simulink library "xblocks_library_pfbs"  (Simulink 7.6)
settings: Solver=ode45  SolverMode=SingleTasking  StartTime=0.0  StopTime=10.0  RelTol=1e-3
libraries: xbsIndex_r4 x151
(part 1 of 2)
settings Model: Creator=mdexter  LastModifiedBy=Glenn

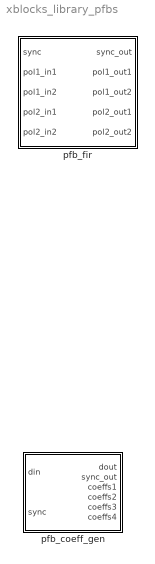
== system xblocks_library_pfbs ==
  pfb_coeff_gen : Subsystem  mask(pfb_coeff_gen){PFBSize=6, CoeffBitWidth=8, TotalTaps=4, CoeffDistMem=0, WindowType=hamming, bram_latency=2, n_inputs=0, nput=0, fwidth=1}
      mask prompts: PFBSize "Size of PFB: (2^? pnts)"; CoeffBitWidth "Bitwidth of Coefficients:"; TotalTaps "Total Number of Taps:"; CoeffDistMem "Implement Coeff Gen in Distributed Memory"; WindowType "Windowing Function:"; bram_latency "BRAM Latency"; n_inputs "Number of Simultaneous Inputs: (2^?)"; nput "This is input number:"; fwidth "Bin Width (normal=1)"
      mask init:
      | config.source = str2func('pfb_coeff_gen_init_xblock');
      | config.toplevel = gcb;
      | config.depend = get_dependlist('pfb_coeff_gen');
      | set_param(gcb,'LinkStatus','inactive');
      | xBlock(config, {config.toplevel, ...
      |     PFBSize, ...
      |     CoeffBitWidth, ...
      |     TotalTaps, ...
      |     CoeffDistMem, ...
      |     WindowType, ...
      |     bram_latency, ...
      |     n_inputs, ...
      |     nput, ...
      |     fwidth});
      settings: AttributesFormatString=PFBSize=6, n_inputs=0, taps=4
  pfb_fir : Subsystem  mask(pfb_fir){PFBSize=5, TotalTaps=2, WindowType=hamming, n_inputs=1, MakeBiplex=on, BitWidthIn=8, BitWidthOut=18, CoeffBitWidth=18, CoeffDistMem=off, add_latency=1, mult_latency=2, bram_latency=2, quantization=Round  (unbiased: +/- Inf), fwidth=1, specify_mult=off, mult_spec=[2                                      2], oversample_factor=0, oversample_index=0}
      mask prompts: PFBSize "Size of PFB: (2^? pnts)"; TotalTaps "Total Number of Taps:"; WindowType "Windowing Function:"; n_inputs "Number of Simultaneous Inputs: (2^?)"; MakeBiplex "Make Biplex"; BitWidthIn "Input Bitwidth:"; BitWidthOut "Output Bitwidth:"; CoeffBitWidth "Coefficient Bitwidth:"; CoeffDistMem "Use Distributed Memory for Coeffs"; add_latency "Add Latency"; mult_latency "Mult Latency"; bram_latency "BRAM Latency"; quantization "Quantization Behavior"; fwidth "Bin Width Scaling (normal=1)"; specify_mult "Specify multiplier use (behavioral if not specified)"; mult_spec "Multiplier specification (0=core, 1=embedded, 2=behavioural) (left=1st tap)"; oversample_factor "Oversample factor (normal=1)"; oversample_index "Oversample index (0 upto oversample factor)"
      mask init:
      | config.source = str2func('pfb_fir_init_xblock');
      | config.toplevel = gcb;
      | config.depend = get_dependlist('pfb_fir');
      | set_param(gcb,'LinkStatus','inactive');
      | xBlock(config,{config.toplevel, ...
      |     'PFBSize', PFBSize, ...
      |     'TotalTaps', TotalTaps, ...
      |     'WindowType', WindowType, ...
      |     'n_inputs', n_inputs, ...
      |     'MakeBiplex', MakeBiplex, ...
      |     'BitWidthIn', BitWidthIn, ...
      |     'BitWidthOut', BitWidthOut, ...
      |     'CoeffBitWidth', CoeffBitWidth, ...
      |     'CoeffDistMem', CoeffDistMem, ...
      |     'add_latency', add_latency, ...
      |     'mult_latency', mult_latency, ...
      |     'bram_latency', bram_latency, ...
      |     'quantization', quantization, ...
      |     'fwidth', fwidth,...
      |     'specify_mult', specify_mult,...
      |     'mult_spec', mult_spec,...
      |     'oversample_factor', oversample_factor,...
      |     'oversample_index', oversample_index});
      settings: AttributesFormatString=taps=2, add_latency=1
      mask Help: eval('xlWeb(''http://casper.berkeley.edu/wiki/Pfb_fir'')')
      mask StyleString: edit,edit,popup(bartlett|barthannwin|blackman|blackmanharris|bohamwin|chebwin|flattopwin|gausswin|hamming|hann|kaiser|nuttallwin|parzenwin|rectwin|tukeywin|triang|userwindow),edit,checkbox,edit,edit,edit,checkbox,edit,edit,edit,popup(Truncate|Round  (unbiased: +/- Inf)|Round  (unbiased: Even Values)),edit,checkbox,edit,edit,edit
      mask CallbackString:
      | |%num_taps = eval(get_param(gcb, 'TotalTaps'));
      | %old_vec = eval(get_param(gcb, 'mult_spec'));
      | 
      | %vec = 2.*ones(1,num_taps);
      | %old_size = length(old_vec);
      | 
      | %if(old_size <= num_taps),
      | %   new_size = old_size;
      | %else,
      | %    new_size = num_taps;
      | %end
      | 
      | %for n = 1:new_size, vec(n) = old_vec(n); end
      | %set_param(gcb, 'mult_spec', mat2str(vec));||||||||||||%num_taps = eval(get_param(gcb, 'TotalTaps'));
      | %old_vec = eval(get_param(gcb, 'mult_spec'));
      | 
      | %vec = 2.*ones(1,num_taps);
      | %old_size = length(old_vec);
      | 
      | %if(old_size <= num_taps),
      | %    new_size = old_size;
      | %else,
      | %    new_size = num_taps;
      | %end
      | 
      | %for n = 1:new_size, vec(n) = old_vec(n); end
      | %set_param(gcb, 'mult_spec', mat2str(vec));|%specify_mult = get_param(gcb,'specify_mult');
      | %if( strcmp(specify_mult,'off')),
      | %    set_param(gcb, 'MaskEnables', {'on','on','on','on','on','on','on','on','on','on','on','on','on','on','on','off'});
      | %else
      | %    set_param(gcb, 'MaskEnables', {'on','on','on','on','on','on','on','on','on','on','on','on','on','on','on','on'});
      | %end
      | 
      | |%specify_mult = get_param(gcb,'specify_mult');
      | %if( strcmp(specify_mult,'off')),
      | %    set_param(gcb, 'MaskEnables', {'on','on','on','on','on','on','on','on','on','on','on','on','on','on','on','off'});
      | %else
      | %    set_param(gcb, 'MaskEnables', {'on','on','on','on','on','on','on','on','on','on','on','on','on','on','on','on'});
      | %end
      | 
      | ||

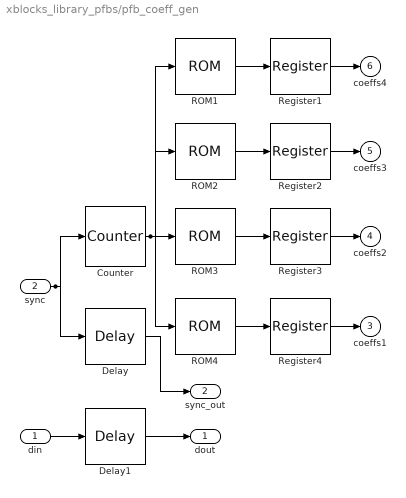
== system xblocks_library_pfbs/pfb_coeff_gen ==
  din : Inport
  sync : Inport  Port=2
  Counter : xbsIndex_r4/Counter  cnt_type=Free Running  cnt_to=Inf  operation=Up  start_count=0  cnt_by_val=1  arith_type=Unsigned  n_bits=6  bin_pt=0  load_pin=off  rst=on  en=off  explicit_period=on  period=1  dbl_ovrd=off  use_behavioral_HDL=off  implementation=Fabric  use_rpm=on  block_type=counter
  Delay : xbsIndex_r4/Delay  en=off  latency=3  dbl_ovrd=off  reg_retiming=off  block_type=delay
  Delay1 : xbsIndex_r4/Delay  en=off  latency=3  dbl_ovrd=off  reg_retiming=off  block_type=delay
  ROM1 : xbsIndex_r4/ROM  depth=64  initVector=[-3.1185374660155e-018 -0.000630767340734862 -0.00127665235543742 -0.00194310743224035 -0.00263564676491746 -0.00335979233260294 -0.00412101838978196 -0.00492469476174935 -0.00577602925112446 -0.00668000946994591 -0.0076413444192915 -0.00866440614422574 -0.00975317179612738 -0.010911166437057 -0.0121414069217606 -0.0134463471921525 -0.0148278253166674 -0.0162870126027097 -0.0178243651045739 -0.0194395778416632 -0.0211315420326285 -0.022898305640208 -0.0247370375091149 -0.0266439953653345 -0.0286144979297191 -0.0306429013818577 -0.0327225803919297 -0.0348459139186967 -0.0370042759510287 -0.039188031348495 -0.0413865369136648 -0.0435881478049666 -0.0457802293743504 -0.0479491744886968 -0.0500804263680376 -0.0521585069473131 -0.0541670507417091 -0.0560888441687308 -0.0579058702531857 -0.0595993586143156 -0.0611498406075495 -0.0625372094668812 -0.0637407852678391 -0.0647393845055283 -0.0655113940574241 -0.0660348492765973 -0.0662875159379727 -0.0662469757381941 -0.0658907150287818 -0.0651962164426562 -0.0641410530558401 -0.0627029847093632 -0.0608600561011471 -0.0585906962440446 -0.0558738188743138 -0.0526889233846958 -0.0490161958479985 -0.0448366096907167 -0.0401320255717928 -0.0348852900191694 -0.0290803323763385 -0.0227022596126709 -0.0157374485549124 -0.00817363510287419]  distributed_mem=Block RAM  rst=off  init_reg=0  en=off  latency=2  arith_type="Signed  (2's comp)"  n_bits=8  bin_pt=7  dbl_ovrd=off  optimize=Area  use_rpm=on  block_type=sprom
  ROM2 : xbsIndex_r4/ROM  depth=64  initVector=[2.11605855357879e-017 0.00879274926085128 0.0182123008044376 0.0282646654074538 0.038954108579165 0.0502830880501052 0.0622521970115558 0.0748601134277915 0.0881035557207456 0.101977245102897 0.116473874808906 0.131584086449929 0.147296453686772 0.16359747338912 0.180471564418265 0.197901074140048 0.215866292743331 0.234345475407368 0.253314872329023 0.272748766588106 0.29261951979626 0.312897625441996 0.333551769811778 0.354548900334662 0.375854301166013 0.39743167579445 0.419243236425489 0.441249799865535 0.463410889601092 0.485684843740308 0.508028928457608 0.530399456557046 0.552751910746464 0.575041071192575 0.597221146906817 0.619245910493353 0.641068835774032 0.662643237790492 0.683922414671039 0.704859790839448 0.725409061034526 0.745524334603159 0.765160279525672 0.784272265630716 0.802816506457524 0.820750199226298 0.838031662382672 0.854620470189629 0.870477583849913 0.885565478653822 0.899848266661255 0.91329181444297 0.925863855424124 0.937534096393168 0.948274317761146 0.958058467180069 0.966862746154448 0.974665689306961 0.981448235987612 0.987193793945478 0.99188829481302 0.995520241184955 0.998080745106585 0.99956355782024]  distributed_mem=Block RAM  rst=off  init_reg=0  en=off  latency=2  arith_type="Signed  (2's comp)"  n_bits=8  bin_pt=7  dbl_ovrd=off  optimize=Area  use_rpm=on  block_type=sprom
  ROM3 : xbsIndex_r4/ROM  depth=64  initVector=[0.999965090652822 0.99928442696235 0.99752332509661 0.994686212352466 0.990780169959861 0.985814909149891 0.979802738401511 0.972758521996084 0.964699630043176 0.955645880174459 0.945619471135172 0.934644908534211 0.922748923044456 0.909960381374135 0.89631019035795 0.881831194543024 0.866558067669544 0.850527198468991 0.83377657122414 0.816345641554348 0.798275207907048 0.779607279251688 0.760384939485607 0.740652209072382 0.720453904442071 0.699835495689393 0.678842963110256 0.657522653119166 0.635921134089847 0.614085052658984 0.592060991028308 0.569895325793337 0.547634088817976 0.525322830662984 0.503006487062978 0.480729248931329 0.458534436355056 0.436464377022686 0.414560289507162 0.39286217180335 0.371408695495545 0.350237105904836 0.329383128539273 0.308880882141693 0.288762798600841 0.269059549961341 0.249799982737069 0.231011059700927 0.212717809291838 0.194943282747282 0.177708519036935 0.161032517640107 0.144932219176911 0.129422493870459 0.114516137785164 0.100223876754423 0.0865543778798294 0.0735142684536453 0.0611081621267689 0.0493386921159191 0.0382065512163987 0.0277105383606731 0.0178476114382339 0.0086129460689059]  distributed_mem=Block RAM  rst=off  init_reg=0  en=off  latency=2  arith_type="Signed  (2's comp)"  n_bits=8  bin_pt=7  dbl_ovrd=off  optimize=Area  use_rpm=on  block_type=sprom
  ROM4 : xbsIndex_r4/ROM  depth=64  initVector=[2.07187717402902e-017 -0.00799941722240988 -0.0153950696762068 -0.0221982159646857 -0.0284215259962463 -0.0340789940546858 -0.0391858485833677 -0.0437584591154741 -0.0478142407894676 -0.0513715568937888 -0.0544496198876778 -0.0570683913458442 -0.0592484812735286 -0.0610110472353188 -0.0623776937359413 -0.0633703722841764 -0.0640112825620935 -0.0643227751110339 -0.0643272559332322 -0.0640470933937545 -0.0635045277916038 -0.0627215839515021 -0.0617199871690848 -0.0605210828221477 -0.0591457599392603 -0.0576143789946302 -0.0559467041746632 -0.0541618403373513 -0.0522781748605462 -0.0503133245494637 -0.0482840877475476 -0.0462064017682173 -0.0440953057381763 -0.0419649089159751 -0.0398283645225593 -0.0376978490936883 -0.0355845473375377 -0.0334986424546007 -0.0314493118513142 -0.0294447281537699 -0.0274920654035405 -0.0255975102941681 -0.023766278284333 -0.0220026344022442 -0.0203099185354575 -0.0186905749812331 -0.017146186014759 -0.0156775092161722 -0.0142845182823737 -0.0129664470362087 -0.01172183633373 -0.0105485835600183 -0.00944399439543556 -0.0084048365272635 -0.00742739497645097 -0.0065075287056645 -0.00564072817301709 -0.00482217349572776 -0.00404679288952885 -0.00330932105286414 -0.00260435716978029 -0.00192642221186661 -0.00127001522759956 -0.000629668316944681]  distributed_mem=Block RAM  rst=off  init_reg=0  en=off  latency=2  arith_type="Signed  (2's comp)"  n_bits=8  bin_pt=7  dbl_ovrd=off  optimize=Area  use_rpm=on  block_type=sprom
  Register{1..4} (4 alike) : xbsIndex_r4/Register  init=0  rst=off  en=off  dbl_ovrd=off  block_type=register
  dout : Outport
  sync_out : Outport  Port=2
  coeffs1 : Outport  Port=3
  coeffs2 : Outport  Port=4
  coeffs3 : Outport  Port=5
  coeffs4 : Outport  Port=6
  wires:
  sync/1 -> Delay/1, Counter/1
  Counter/1 -> ROM1/1, ROM2/1, ROM3/1, ROM4/1
  Register1/1 -> coeffs4/1
  ROM1/1 -> Register1/1
  Register2/1 -> coeffs3/1
  ROM2/1 -> Register2/1
  Register3/1 -> coeffs2/1
  ROM3/1 -> Register3/1
  Register4/1 -> coeffs1/1
  ROM4/1 -> Register4/1
  Delay1/1 -> dout/1
  din/1 -> Delay1/1
  Delay/1 -> sync_out/1

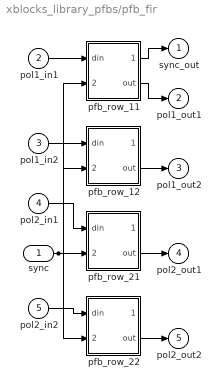
== system xblocks_library_pfbs/pfb_fir ==
  sync : Inport
  pol1_in1 : Inport  Port=2
  pol1_in2 : Inport  Port=3
  pol2_in1 : Inport  Port=4
  pol2_in2 : Inport  Port=5
  pfb_row_11 : Subsystem
  pfb_row_12 : Subsystem
  pfb_row_21 : Subsystem
  pfb_row_22 : Subsystem
  sync_out : Outport
  pol1_out1 : Outport  Port=2
  pol1_out2 : Outport  Port=3
  pol2_out1 : Outport  Port=4
  pol2_out2 : Outport  Port=5
  wires:
  sync/1 -> pfb_row_22/2(sync), pfb_row_21/2(sync), pfb_row_12/2(sync), pfb_row_11/2(sync)
  pfb_row_22/2(out) -> pol2_out2/1
  pol2_in2/1 -> pfb_row_22/1(din)
  pfb_row_21/2(out) -> pol2_out1/1
  pol2_in1/1 -> pfb_row_21/1(din)
  pfb_row_12/2(out) -> pol1_out2/1
  pol1_in2/1 -> pfb_row_12/1(din)
  pfb_row_11/2(out) -> pol1_out1/1
  pfb_row_11/1(sync_out) -> sync_out/1
  pol1_in1/1 -> pfb_row_11/1(din)

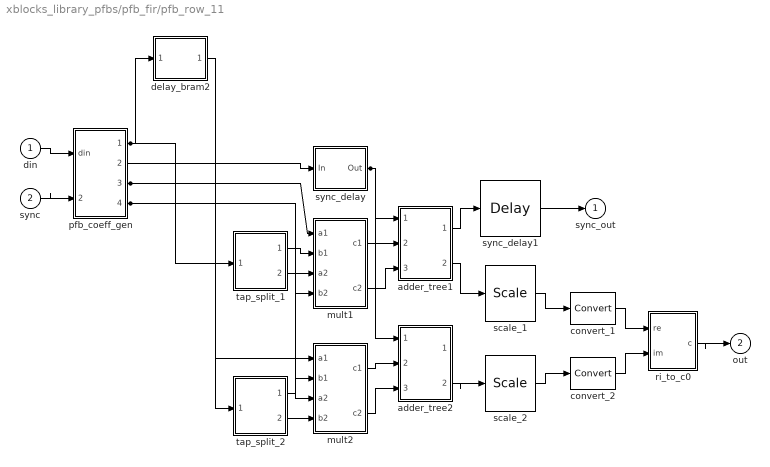
== system xblocks_library_pfbs/pfb_fir/pfb_row_11 ==
  din : Inport
  sync : Inport  Port=2
  adder_tree1 : Subsystem
  adder_tree2 : Subsystem
  convert_1 : xbsIndex_r4/Convert  arith_type="Signed  (2's comp)"  n_bits=18  bin_pt=17  quantization="Round  (unbiased: +/- Inf)"  overflow=Saturate  en=off  latency=2  dbl_ovrd=off  pipeline=on  block_type=convert
  convert_2 : xbsIndex_r4/Convert  arith_type="Signed  (2's comp)"  n_bits=18  bin_pt=17  quantization="Round  (unbiased: +/- Inf)"  overflow=Saturate  en=off  latency=2  dbl_ovrd=off  pipeline=on  block_type=convert
  delay_bram2 : Subsystem
  mult1 : Subsystem
  mult2 : Subsystem
  pfb_coeff_gen : Subsystem
      settings: AttributesFormatString=PFBSize=5, n_inputs=1, taps=2
  ri_to_c0 : Subsystem
  scale_1 : xbsIndex_r4/Scale  scale_factor=-2  dbl_ovrd=off  block_type=scale
  scale_2 : xbsIndex_r4/Scale  scale_factor=-2  dbl_ovrd=off  block_type=scale
  sync_delay : Subsystem
  sync_delay1 : xbsIndex_r4/Delay  en=off  latency=2  dbl_ovrd=off  reg_retiming=off  block_type=delay
  tap_split_1 : Subsystem
      settings: AttributesFormatString=Fix_8_7
  tap_split_2 : Subsystem
      settings: AttributesFormatString=Fix_8_7
  sync_out : Outport
  out : Outport  Port=2
  wires:
  pfb_coeff_gen/1(dout) -> tap_split_1/1(inport), delay_bram2/1(din_1_1)
  pfb_coeff_gen/3(coeffs1) -> mult2/1(a1), mult1/1(a1)
  pfb_coeff_gen/4(coeffs2) -> mult2/3(a2), mult1/3(a2)
  sync_delay/1(Out) -> adder_tree2/1(sync), adder_tree1/1(sync)
  ri_to_c0/1(c) -> out/1
  convert_2/1 -> ri_to_c0/2(im)
  convert_1/1 -> ri_to_c0/1(re)
  scale_2/1 -> convert_2/1
  adder_tree2/2(dout) -> scale_2/1
  mult2/2(c2) -> adder_tree2/3(din_2)
  mult2/1(c1) -> adder_tree2/2(din_1)
  tap_split_2/2(outport2) -> mult2/4(b2)
  tap_split_1/2(outport2) -> mult2/2(b1)
  sync_delay1/1 -> sync_out/1
  adder_tree1/1(sync_out) -> sync_delay1/1
  scale_1/1 -> convert_1/1
  adder_tree1/2(dout) -> scale_1/1
  mult1/2(c2) -> adder_tree1/3(din_2)
  mult1/1(c1) -> adder_tree1/2(din_1)
  tap_split_2/1(outport1) -> mult1/4(b2)
  tap_split_1/1(outport1) -> mult1/2(b1)
  delay_bram2/1(dout_1_1) -> tap_split_2/1(inport)
  pfb_coeff_gen/2(sync_out) -> sync_delay/1(In)
  sync/1 -> pfb_coeff_gen/2(sync)
  din/1 -> pfb_coeff_gen/1(din)

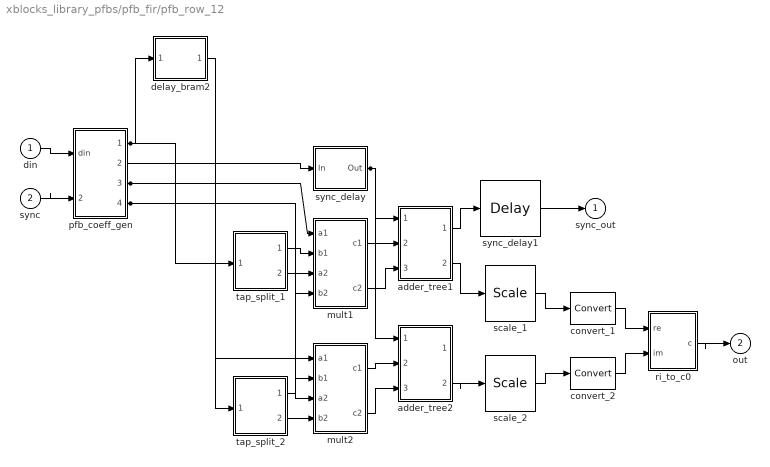
== system xblocks_library_pfbs/pfb_fir/pfb_row_12 ==
  din : Inport
  sync : Inport  Port=2
  adder_tree1 : Subsystem
  adder_tree2 : Subsystem
  convert_1 : xbsIndex_r4/Convert  arith_type="Signed  (2's comp)"  n_bits=18  bin_pt=17  quantization="Round  (unbiased: +/- Inf)"  overflow=Saturate  en=off  latency=2  dbl_ovrd=off  pipeline=on  block_type=convert
  convert_2 : xbsIndex_r4/Convert  arith_type="Signed  (2's comp)"  n_bits=18  bin_pt=17  quantization="Round  (unbiased: +/- Inf)"  overflow=Saturate  en=off  latency=2  dbl_ovrd=off  pipeline=on  block_type=convert
  delay_bram2 : Subsystem
  mult1 : Subsystem
  mult2 : Subsystem
  pfb_coeff_gen : Subsystem
      settings: AttributesFormatString=PFBSize=5, n_inputs=1, taps=2
  ri_to_c0 : Subsystem
  scale_1 : xbsIndex_r4/Scale  scale_factor=-2  dbl_ovrd=off  block_type=scale
  scale_2 : xbsIndex_r4/Scale  scale_factor=-2  dbl_ovrd=off  block_type=scale
  sync_delay : Subsystem
  sync_delay1 : xbsIndex_r4/Delay  en=off  latency=2  dbl_ovrd=off  reg_retiming=off  block_type=delay
  tap_split_1 : Subsystem
      settings: AttributesFormatString=Fix_8_7
  tap_split_2 : Subsystem
      settings: AttributesFormatString=Fix_8_7
  sync_out : Outport
  out : Outport  Port=2
  wires:
  pfb_coeff_gen/1(dout) -> tap_split_1/1(inport), delay_bram2/1(din_1_1)
  pfb_coeff_gen/3(coeffs1) -> mult2/1(a1), mult1/1(a1)
  pfb_coeff_gen/4(coeffs2) -> mult2/3(a2), mult1/3(a2)
  sync_delay/1(Out) -> adder_tree2/1(sync), adder_tree1/1(sync)
  ri_to_c0/1(c) -> out/1
  convert_2/1 -> ri_to_c0/2(im)
  convert_1/1 -> ri_to_c0/1(re)
  scale_2/1 -> convert_2/1
  adder_tree2/2(dout) -> scale_2/1
  mult2/2(c2) -> adder_tree2/3(din_2)
  mult2/1(c1) -> adder_tree2/2(din_1)
  tap_split_2/2(outport2) -> mult2/4(b2)
  tap_split_1/2(outport2) -> mult2/2(b1)
  sync_delay1/1 -> sync_out/1
  adder_tree1/1(sync_out) -> sync_delay1/1
  scale_1/1 -> convert_1/1
  adder_tree1/2(dout) -> scale_1/1
  mult1/2(c2) -> adder_tree1/3(din_2)
  mult1/1(c1) -> adder_tree1/2(din_1)
  tap_split_2/1(outport1) -> mult1/4(b2)
  tap_split_1/1(outport1) -> mult1/2(b1)
  delay_bram2/1(dout_1_1) -> tap_split_2/1(inport)
  pfb_coeff_gen/2(sync_out) -> sync_delay/1(In)
  sync/1 -> pfb_coeff_gen/2(sync)
  din/1 -> pfb_coeff_gen/1(din)

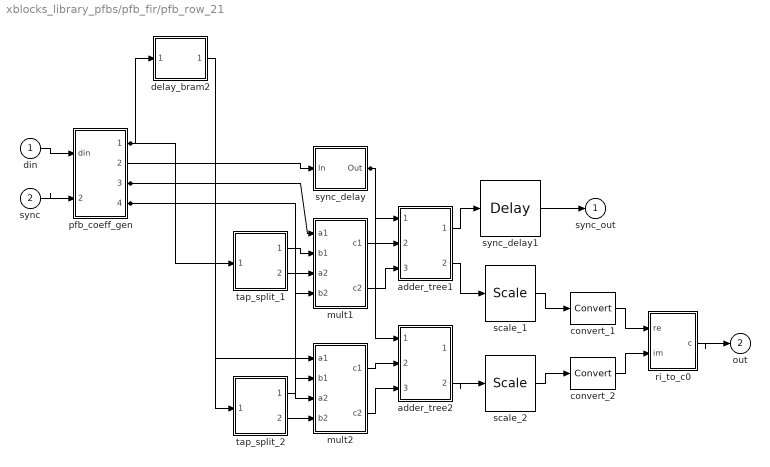
== system xblocks_library_pfbs/pfb_fir/pfb_row_21 ==
  din : Inport
  sync : Inport  Port=2
  adder_tree1 : Subsystem
  adder_tree2 : Subsystem
  convert_1 : xbsIndex_r4/Convert  arith_type="Signed  (2's comp)"  n_bits=18  bin_pt=17  quantization="Round  (unbiased: +/- Inf)"  overflow=Saturate  en=off  latency=2  dbl_ovrd=off  pipeline=on  block_type=convert
  convert_2 : xbsIndex_r4/Convert  arith_type="Signed  (2's comp)"  n_bits=18  bin_pt=17  quantization="Round  (unbiased: +/- Inf)"  overflow=Saturate  en=off  latency=2  dbl_ovrd=off  pipeline=on  block_type=convert
  delay_bram2 : Subsystem
  mult1 : Subsystem
  mult2 : Subsystem
  pfb_coeff_gen : Subsystem
      settings: AttributesFormatString=PFBSize=5, n_inputs=1, taps=2
  ri_to_c0 : Subsystem
  scale_1 : xbsIndex_r4/Scale  scale_factor=-2  dbl_ovrd=off  block_type=scale
  scale_2 : xbsIndex_r4/Scale  scale_factor=-2  dbl_ovrd=off  block_type=scale
  sync_delay : Subsystem
  sync_delay1 : xbsIndex_r4/Delay  en=off  latency=2  dbl_ovrd=off  reg_retiming=off  block_type=delay
  tap_split_1 : Subsystem
      settings: AttributesFormatString=Fix_8_7
  tap_split_2 : Subsystem
      settings: AttributesFormatString=Fix_8_7
  sync_out : Outport
  out : Outport  Port=2
  wires:
  pfb_coeff_gen/1(dout) -> tap_split_1/1(inport), delay_bram2/1(din_1_1)
  pfb_coeff_gen/3(coeffs1) -> mult2/1(a1), mult1/1(a1)
  pfb_coeff_gen/4(coeffs2) -> mult2/3(a2), mult1/3(a2)
  sync_delay/1(Out) -> adder_tree2/1(sync), adder_tree1/1(sync)
  ri_to_c0/1(c) -> out/1
  convert_2/1 -> ri_to_c0/2(im)
  convert_1/1 -> ri_to_c0/1(re)
  scale_2/1 -> convert_2/1
  adder_tree2/2(dout) -> scale_2/1
  mult2/2(c2) -> adder_tree2/3(din_2)
  mult2/1(c1) -> adder_tree2/2(din_1)
  tap_split_2/2(outport2) -> mult2/4(b2)
  tap_split_1/2(outport2) -> mult2/2(b1)
  sync_delay1/1 -> sync_out/1
  adder_tree1/1(sync_out) -> sync_delay1/1
  scale_1/1 -> convert_1/1
  adder_tree1/2(dout) -> scale_1/1
  mult1/2(c2) -> adder_tree1/3(din_2)
  mult1/1(c1) -> adder_tree1/2(din_1)
  tap_split_2/1(outport1) -> mult1/4(b2)
  tap_split_1/1(outport1) -> mult1/2(b1)
  delay_bram2/1(dout_1_1) -> tap_split_2/1(inport)
  pfb_coeff_gen/2(sync_out) -> sync_delay/1(In)
  sync/1 -> pfb_coeff_gen/2(sync)
  din/1 -> pfb_coeff_gen/1(din)

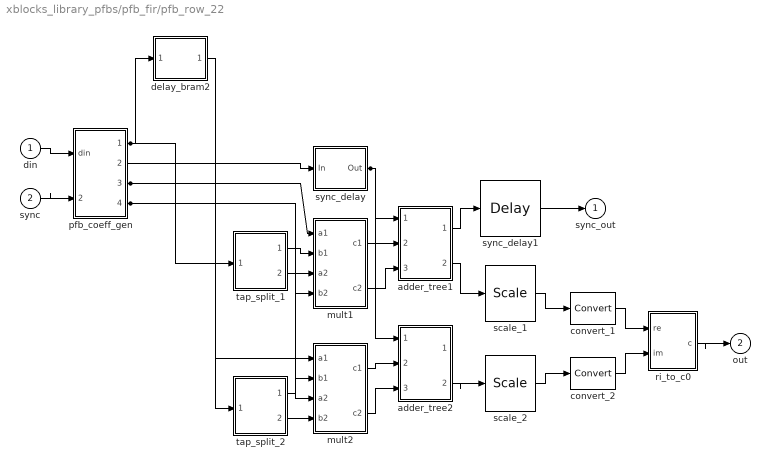
== system xblocks_library_pfbs/pfb_fir/pfb_row_22 ==
  din : Inport
  sync : Inport  Port=2
  adder_tree1 : Subsystem
  adder_tree2 : Subsystem
  convert_1 : xbsIndex_r4/Convert  arith_type="Signed  (2's comp)"  n_bits=18  bin_pt=17  quantization="Round  (unbiased: +/- Inf)"  overflow=Saturate  en=off  latency=2  dbl_ovrd=off  pipeline=on  block_type=convert
  convert_2 : xbsIndex_r4/Convert  arith_type="Signed  (2's comp)"  n_bits=18  bin_pt=17  quantization="Round  (unbiased: +/- Inf)"  overflow=Saturate  en=off  latency=2  dbl_ovrd=off  pipeline=on  block_type=convert
  delay_bram2 : Subsystem
  mult1 : Subsystem
  mult2 : Subsystem
  pfb_coeff_gen : Subsystem
      settings: AttributesFormatString=PFBSize=5, n_inputs=1, taps=2
  ri_to_c0 : Subsystem
  scale_1 : xbsIndex_r4/Scale  scale_factor=-2  dbl_ovrd=off  block_type=scale
  scale_2 : xbsIndex_r4/Scale  scale_factor=-2  dbl_ovrd=off  block_type=scale
  sync_delay : Subsystem
  sync_delay1 : xbsIndex_r4/Delay  en=off  latency=2  dbl_ovrd=off  reg_retiming=off  block_type=delay
  tap_split_1 : Subsystem
      settings: AttributesFormatString=Fix_8_7
  tap_split_2 : Subsystem
      settings: AttributesFormatString=Fix_8_7
  sync_out : Outport
  out : Outport  Port=2
  wires:
  pfb_coeff_gen/1(dout) -> tap_split_1/1(inport), delay_bram2/1(din_1_1)
  pfb_coeff_gen/3(coeffs1) -> mult2/1(a1), mult1/1(a1)
  pfb_coeff_gen/4(coeffs2) -> mult2/3(a2), mult1/3(a2)
  sync_delay/1(Out) -> adder_tree2/1(sync), adder_tree1/1(sync)
  ri_to_c0/1(c) -> out/1
  convert_2/1 -> ri_to_c0/2(im)
  convert_1/1 -> ri_to_c0/1(re)
  scale_2/1 -> convert_2/1
  adder_tree2/2(dout) -> scale_2/1
  mult2/2(c2) -> adder_tree2/3(din_2)
  mult2/1(c1) -> adder_tree2/2(din_1)
  tap_split_2/2(outport2) -> mult2/4(b2)
  tap_split_1/2(outport2) -> mult2/2(b1)
  sync_delay1/1 -> sync_out/1
  adder_tree1/1(sync_out) -> sync_delay1/1
  scale_1/1 -> convert_1/1
  adder_tree1/2(dout) -> scale_1/1
  mult1/2(c2) -> adder_tree1/3(din_2)
  mult1/1(c1) -> adder_tree1/2(din_1)
  tap_split_2/1(outport1) -> mult1/4(b2)
  tap_split_1/1(outport1) -> mult1/2(b1)
  delay_bram2/1(dout_1_1) -> tap_split_2/1(inport)
  pfb_coeff_gen/2(sync_out) -> sync_delay/1(In)
  sync/1 -> pfb_coeff_gen/2(sync)
  din/1 -> pfb_coeff_gen/1(din)

== system xblocks_library_pfbs/pfb_fir/pfb_row_11/adder_tree1 ==
  sync : Inport
  din_1 : Inport  Port=2
  din_2 : Inport  Port=3
  adder_0 : xbsIndex_r4/AddSub  mode=Addition  use_carryin=off  use_carryout=off  en=off  latency=1  precision=Full  arith_type=Unsigned  n_bits=18  bin_pt=17  quantization="Round  (unbiased: +/- Inf)"  overflow=Wrap  dbl_ovrd=off  use_behavioral_HDL=on  hw_selection=Fabric  pipelined=off  block_type=addsub
  sync_delay : xbsIndex_r4/Delay  en=off  latency=1  dbl_ovrd=off  reg_retiming=off  block_type=delay
  sync_out : Outport
  dout : Outport  Port=2
  wires:
  adder_0/1 -> dout/1
  din_1/1 -> adder_0/2
  din_2/1 -> adder_0/1
  sync_delay/1 -> sync_out/1
  sync/1 -> sync_delay/1

== system xblocks_library_pfbs/pfb_fir/pfb_row_11/adder_tree2 ==
  sync : Inport
  din_1 : Inport  Port=2
  din_2 : Inport  Port=3
  adder_0 : xbsIndex_r4/AddSub  mode=Addition  use_carryin=off  use_carryout=off  en=off  latency=1  precision=Full  arith_type=Unsigned  n_bits=18  bin_pt=17  quantization="Round  (unbiased: +/- Inf)"  overflow=Wrap  dbl_ovrd=off  use_behavioral_HDL=on  hw_selection=Fabric  pipelined=off  block_type=addsub
  sync_delay : xbsIndex_r4/Delay  en=off  latency=1  dbl_ovrd=off  reg_retiming=off  block_type=delay
  sync_out : Outport
  dout : Outport  Port=2
  wires:
  adder_0/1 -> dout/1
  din_1/1 -> adder_0/2
  din_2/1 -> adder_0/1
  sync_delay/1 -> sync_out/1
  sync/1 -> sync_delay/1

== system xblocks_library_pfbs/pfb_fir/pfb_row_11/delay_bram2 ==
  din_1_1 : Inport
  Constant2 : xbsIndex_r4/Constant  arith_type=Boolean  const=1  n_bits=1  bin_pt=0  explicit_period=on  period=1  equ=P=C  opselect=C  inp2=PCIN>>17  opr=+  inp1=P  carry=CIN  dbl_ovrd=off  block_type=constant
  Counter : xbsIndex_r4/Counter  cnt_type=Count Limited  cnt_to=2  operation=Up  start_count=0  cnt_by_val=1  arith_type=Unsigned  n_bits=3  bin_pt=0  load_pin=off  rst=off  en=off  explicit_period=on  period=1  dbl_ovrd=off  use_behavioral_HDL=off  implementation=Fabric  use_rpm=0  block_type=counter
  bram1 : xbsIndex_r4/Single Port RAM  depth=8  initVector=0  distributed_mem=Block RAM  write_mode=Read Before Write  rst=off  init_reg=0  en=off  latency=4  dbl_ovrd=off  optimize=Area  use_rpm=off  block_type=spram
  dout_1_1 : Outport
  wires:
  bram1/1 -> dout_1_1/1
  Constant2/1 -> bram1/3
  din_1_1/1 -> bram1/2
  Counter/1 -> bram1/1

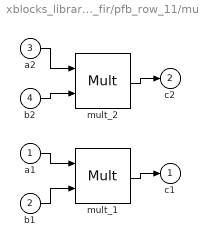
== system xblocks_library_pfbs/pfb_fir/pfb_row_11/mult1 ==
  a1 : Inport
  b1 : Inport  Port=2
  a2 : Inport  Port=3
  b2 : Inport  Port=4
  mult_1 : xbsIndex_r4/Mult  precision=Full  arith_type="Signed  (2's comp)"  n_bits=16  bin_pt=14  quantization=Truncate  overflow=Wrap  en=off  latency=2  dbl_ovrd=off  use_behavioral_HDL=off  opt=Speed  use_embedded=on  optimum_pipeline=off  pipeline=on  use_rpm=on  placement_style=Triangular  block_type=mult
  mult_2 : xbsIndex_r4/Mult  precision=Full  arith_type="Signed  (2's comp)"  n_bits=16  bin_pt=14  quantization=Truncate  overflow=Wrap  en=off  latency=2  dbl_ovrd=off  use_behavioral_HDL=off  opt=Speed  use_embedded=on  optimum_pipeline=off  pipeline=on  use_rpm=on  placement_style=Triangular  block_type=mult
  c1 : Outport
  c2 : Outport  Port=2
  wires:
  mult_2/1 -> c2/1
  b2/1 -> mult_2/2
  a2/1 -> mult_2/1
  mult_1/1 -> c1/1
  b1/1 -> mult_1/2
  a1/1 -> mult_1/1

== system xblocks_library_pfbs/pfb_fir/pfb_row_11/mult2 ==
  a1 : Inport
  b1 : Inport  Port=2
  a2 : Inport  Port=3
  b2 : Inport  Port=4
  mult_1 : xbsIndex_r4/Mult  precision=Full  arith_type="Signed  (2's comp)"  n_bits=16  bin_pt=14  quantization=Truncate  overflow=Wrap  en=off  latency=2  dbl_ovrd=off  use_behavioral_HDL=off  opt=Speed  use_embedded=on  optimum_pipeline=off  pipeline=on  use_rpm=on  placement_style=Triangular  block_type=mult
  mult_2 : xbsIndex_r4/Mult  precision=Full  arith_type="Signed  (2's comp)"  n_bits=16  bin_pt=14  quantization=Truncate  overflow=Wrap  en=off  latency=2  dbl_ovrd=off  use_behavioral_HDL=off  opt=Speed  use_embedded=on  optimum_pipeline=off  pipeline=on  use_rpm=on  placement_style=Triangular  block_type=mult
  c1 : Outport
  c2 : Outport  Port=2
  wires:
  mult_2/1 -> c2/1
  b2/1 -> mult_2/2
  a2/1 -> mult_2/1
  mult_1/1 -> c1/1
  b1/1 -> mult_1/2
  a1/1 -> mult_1/1

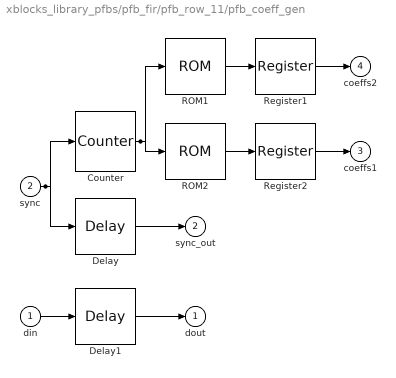
== system xblocks_library_pfbs/pfb_fir/pfb_row_11/pfb_coeff_gen ==
  din : Inport
  sync : Inport  Port=2
  Counter : xbsIndex_r4/Counter  cnt_type=Free Running  cnt_to=Inf  operation=Up  start_count=0  cnt_by_val=1  arith_type=Unsigned  n_bits=4  bin_pt=0  load_pin=off  rst=on  en=off  explicit_period=on  period=1  dbl_ovrd=off  use_behavioral_HDL=off  implementation=Fabric  use_rpm=on  block_type=counter
  Delay : xbsIndex_r4/Delay  en=off  latency=3  dbl_ovrd=off  reg_retiming=off  block_type=delay
  Delay1 : xbsIndex_r4/Delay  en=off  latency=3  dbl_ovrd=off  reg_retiming=off  block_type=delay
  ROM1 : xbsIndex_r4/ROM  depth=16  initVector=[3.1185374660155e-018 0.00590327410394983 0.0161656170740572 0.0348093655963705 0.0656663902623872 0.111805550739839 0.175009649863286 0.255372651705337 0.351075507876153 0.458378509738419 0.571842120148991 0.684759989924505 0.789760948691871 0.879514682510877 0.947461498288465 0.988481980811812]  distributed_mem=Block RAM  rst=off  init_reg=0  en=off  latency=2  arith_type="Signed  (2's comp)"  n_bits=18  bin_pt=17  dbl_ovrd=off  optimize=Area  use_rpm=on  block_type=sprom
  ROM2 : xbsIndex_r4/ROM  depth=16  initVector=[0.999428183760704 0.979453626314143 0.930102884263783 0.855150032153279 0.760205026373763 0.652134554227596 0.538365459275223 0.426151900540966 0.321890335701215 0.230558971056803 0.155341565541388 0.0974716688563325 0.0563056492152491 0.0296048151953255 0.0139821303092272 0.00545054213132689]  distributed_mem=Block RAM  rst=off  init_reg=0  en=off  latency=2  arith_type="Signed  (2's comp)"  n_bits=18  bin_pt=17  dbl_ovrd=off  optimize=Area  use_rpm=on  block_type=sprom
  Register1 : xbsIndex_r4/Register  init=0  rst=off  en=off  dbl_ovrd=off  block_type=register
  Register2 : xbsIndex_r4/Register  init=0  rst=off  en=off  dbl_ovrd=off  block_type=register
  dout : Outport
  sync_out : Outport  Port=2
  coeffs1 : Outport  Port=3
  coeffs2 : Outport  Port=4
  wires:
  sync/1 -> Delay/1, Counter/1
  Counter/1 -> ROM1/1, ROM2/1
  Register1/1 -> coeffs2/1
  ROM1/1 -> Register1/1
  Register2/1 -> coeffs1/1
  ROM2/1 -> Register2/1
  Delay1/1 -> dout/1
  din/1 -> Delay1/1
  Delay/1 -> sync_out/1

== system xblocks_library_pfbs/pfb_fir/pfb_row_11/ri_to_c0 ==
  re : Inport
  im : Inport  Port=2
  concat : xbsIndex_r4/Concat  num_inputs=2  dbl_ovrd=off  block_type=concat
  force_im : xbsIndex_r4/Reinterpret  force_arith_type=on  arith_type=Unsigned  force_bin_pt=on  bin_pt=0  block_type=reinterpret
      settings: infoedit="Changes signal type without altering the binary representation.   You can changed the signal between signed and unsigned, and relocate the binary point.<br><br>Hardware notes: In hardware this block costs nothing.<br><br>Example:  Suppose the input is 6 bits wide, signed, with 2 fractional bits, and the output is forced to unsigned with 0 fractional bits.  Then an input of -2.0 (1110.00 in binary 2's complement) becomes an output of 56 (111000 in binary)."
  force_re : xbsIndex_r4/Reinterpret  force_arith_type=on  arith_type=Unsigned  force_bin_pt=on  bin_pt=0  block_type=reinterpret
      settings: infoedit="Changes signal type without altering the binary representation.   You can changed the signal between signed and unsigned, and relocate the binary point.<br><br>Hardware notes: In hardware this block costs nothing.<br><br>Example:  Suppose the input is 6 bits wide, signed, with 2 fractional bits, and the output is forced to unsigned with 0 fractional bits.  Then an input of -2.0 (1110.00 in binary 2's complement) becomes an output of 56 (111000 in binary)."
  c : Outport
  wires:
  force_re/1 -> concat/1
  re/1 -> force_re/1
  force_im/1 -> concat/2
  im/1 -> force_im/1
  concat/1 -> c/1

== system xblocks_library_pfbs/pfb_fir/pfb_row_11/sync_delay ==
  In : Inport
  sync_del : xbsIndex_r4/Delay  en=off  latency=18  dbl_ovrd=off  reg_retiming=off  block_type=delay
  Out : Outport
  wires:
  sync_del/1 -> Out/1
  In/1 -> sync_del/1

== system xblocks_library_pfbs/pfb_fir/pfb_row_11/tap_split_1 ==
  inport : Inport
  Reinterp1 : xbsIndex_r4/Reinterpret  force_arith_type=on  arith_type="Signed  (2's comp)"  force_bin_pt=on  bin_pt=7  block_type=reinterpret
      settings: infoedit="Changes signal type without altering the binary representation.   You can changed the signal between signed and unsigned, and relocate the binary point.<br><br>Hardware notes: In hardware this block costs nothing.<br><br>Example:  Suppose the input is 6 bits wide, signed, with 2 fractional bits, and the output is forced to unsigned with 0 fractional bits.  Then an input of -2.0 (1110.00 in binary 2's complement) becomes an output of 56 (111000 in binary)."
  Reinterp2 : xbsIndex_r4/Reinterpret  force_arith_type=on  arith_type="Signed  (2's comp)"  force_bin_pt=on  bin_pt=7  block_type=reinterpret
      settings: infoedit="Changes signal type without altering the binary representation.   You can changed the signal between signed and unsigned, and relocate the binary point.<br><br>Hardware notes: In hardware this block costs nothing.<br><br>Example:  Suppose the input is 6 bits wide, signed, with 2 fractional bits, and the output is forced to unsigned with 0 fractional bits.  Then an input of -2.0 (1110.00 in binary 2's complement) becomes an output of 56 (111000 in binary)."
  Slice1 : xbsIndex_r4/Slice  nbits=8  boolean_output=off  mode=Upper Bit Location + Width  bit1=-0  base1=MSB of Input  bit0=0  base0=LSB of Input  dbl_ovrd=off  block_type=slice
  Slice2 : xbsIndex_r4/Slice  nbits=8  boolean_output=off  mode=Upper Bit Location + Width  bit1=-8  base1=MSB of Input  bit0=0  base0=LSB of Input  dbl_ovrd=off  block_type=slice
  outport1 : Outport
  outport2 : Outport  Port=2
  wires:
  inport/1 -> Slice2/1, Slice1/1
  Reinterp2/1 -> outport2/1
  Slice2/1 -> Reinterp2/1  "slice_out2"
  Reinterp1/1 -> outport1/1
  Slice1/1 -> Reinterp1/1  "slice_out1"

== system xblocks_library_pfbs/pfb_fir/pfb_row_11/tap_split_2 ==
  inport : Inport
  Reinterp1 : xbsIndex_r4/Reinterpret  force_arith_type=on  arith_type="Signed  (2's comp)"  force_bin_pt=on  bin_pt=7  block_type=reinterpret
      settings: infoedit="Changes signal type without altering the binary representation.   You can changed the signal between signed and unsigned, and relocate the binary point.<br><br>Hardware notes: In hardware this block costs nothing.<br><br>Example:  Suppose the input is 6 bits wide, signed, with 2 fractional bits, and the output is forced to unsigned with 0 fractional bits.  Then an input of -2.0 (1110.00 in binary 2's complement) becomes an output of 56 (111000 in binary)."
  Reinterp2 : xbsIndex_r4/Reinterpret  force_arith_type=on  arith_type="Signed  (2's comp)"  force_bin_pt=on  bin_pt=7  block_type=reinterpret
      settings: infoedit="Changes signal type without altering the binary representation.   You can changed the signal between signed and unsigned, and relocate the binary point.<br><br>Hardware notes: In hardware this block costs nothing.<br><br>Example:  Suppose the input is 6 bits wide, signed, with 2 fractional bits, and the output is forced to unsigned with 0 fractional bits.  Then an input of -2.0 (1110.00 in binary 2's complement) becomes an output of 56 (111000 in binary)."
  Slice1 : xbsIndex_r4/Slice  nbits=8  boolean_output=off  mode=Upper Bit Location + Width  bit1=-0  base1=MSB of Input  bit0=0  base0=LSB of Input  dbl_ovrd=off  block_type=slice
  Slice2 : xbsIndex_r4/Slice  nbits=8  boolean_output=off  mode=Upper Bit Location + Width  bit1=-8  base1=MSB of Input  bit0=0  base0=LSB of Input  dbl_ovrd=off  block_type=slice
  outport1 : Outport
  outport2 : Outport  Port=2
  wires:
  inport/1 -> Slice2/1, Slice1/1
  Reinterp2/1 -> outport2/1
  Slice2/1 -> Reinterp2/1  "slice_out2"
  Reinterp1/1 -> outport1/1
  Slice1/1 -> Reinterp1/1  "slice_out1"

== system xblocks_library_pfbs/pfb_fir/pfb_row_12/adder_tree1 ==
  sync : Inport
  din_1 : Inport  Port=2
  din_2 : Inport  Port=3
  adder_0 : xbsIndex_r4/AddSub  mode=Addition  use_carryin=off  use_carryout=off  en=off  latency=1  precision=Full  arith_type=Unsigned  n_bits=18  bin_pt=17  quantization="Round  (unbiased: +/- Inf)"  overflow=Wrap  dbl_ovrd=off  use_behavioral_HDL=on  hw_selection=Fabric  pipelined=off  block_type=addsub
  sync_delay : xbsIndex_r4/Delay  en=off  latency=1  dbl_ovrd=off  reg_retiming=off  block_type=delay
  sync_out : Outport
  dout : Outport  Port=2
  wires:
  adder_0/1 -> dout/1
  din_1/1 -> adder_0/2
  din_2/1 -> adder_0/1
  sync_delay/1 -> sync_out/1
  sync/1 -> sync_delay/1

== system xblocks_library_pfbs/pfb_fir/pfb_row_12/adder_tree2 ==
  sync : Inport
  din_1 : Inport  Port=2
  din_2 : Inport  Port=3
  adder_0 : xbsIndex_r4/AddSub  mode=Addition  use_carryin=off  use_carryout=off  en=off  latency=1  precision=Full  arith_type=Unsigned  n_bits=18  bin_pt=17  quantization="Round  (unbiased: +/- Inf)"  overflow=Wrap  dbl_ovrd=off  use_behavioral_HDL=on  hw_selection=Fabric  pipelined=off  block_type=addsub
  sync_delay : xbsIndex_r4/Delay  en=off  latency=1  dbl_ovrd=off  reg_retiming=off  block_type=delay
  sync_out : Outport
  dout : Outport  Port=2
  wires:
  adder_0/1 -> dout/1
  din_1/1 -> adder_0/2
  din_2/1 -> adder_0/1
  sync_delay/1 -> sync_out/1
  sync/1 -> sync_delay/1

== system xblocks_library_pfbs/pfb_fir/pfb_row_12/delay_bram2 ==
  din_1_1 : Inport
  Constant2 : xbsIndex_r4/Constant  arith_type=Boolean  const=1  n_bits=1  bin_pt=0  explicit_period=on  period=1  equ=P=C  opselect=C  inp2=PCIN>>17  opr=+  inp1=P  carry=CIN  dbl_ovrd=off  block_type=constant
  Counter : xbsIndex_r4/Counter  cnt_type=Count Limited  cnt_to=2  operation=Up  start_count=0  cnt_by_val=1  arith_type=Unsigned  n_bits=3  bin_pt=0  load_pin=off  rst=off  en=off  explicit_period=on  period=1  dbl_ovrd=off  use_behavioral_HDL=off  implementation=Fabric  use_rpm=0  block_type=counter
  bram1 : xbsIndex_r4/Single Port RAM  depth=8  initVector=0  distributed_mem=Block RAM  write_mode=Read Before Write  rst=off  init_reg=0  en=off  latency=4  dbl_ovrd=off  optimize=Area  use_rpm=off  block_type=spram
  dout_1_1 : Outport
  wires:
  bram1/1 -> dout_1_1/1
  Constant2/1 -> bram1/3
  din_1_1/1 -> bram1/2
  Counter/1 -> bram1/1

== system xblocks_library_pfbs/pfb_fir/pfb_row_12/mult1 ==
  a1 : Inport
  b1 : Inport  Port=2
  a2 : Inport  Port=3
  b2 : Inport  Port=4
  mult_1 : xbsIndex_r4/Mult  precision=Full  arith_type="Signed  (2's comp)"  n_bits=16  bin_pt=14  quantization=Truncate  overflow=Wrap  en=off  latency=2  dbl_ovrd=off  use_behavioral_HDL=off  opt=Speed  use_embedded=on  optimum_pipeline=off  pipeline=on  use_rpm=on  placement_style=Triangular  block_type=mult
  mult_2 : xbsIndex_r4/Mult  precision=Full  arith_type="Signed  (2's comp)"  n_bits=16  bin_pt=14  quantization=Truncate  overflow=Wrap  en=off  latency=2  dbl_ovrd=off  use_behavioral_HDL=off  opt=Speed  use_embedded=on  optimum_pipeline=off  pipeline=on  use_rpm=on  placement_style=Triangular  block_type=mult
  c1 : Outport
  c2 : Outport  Port=2
  wires:
  mult_2/1 -> c2/1
  b2/1 -> mult_2/2
  a2/1 -> mult_2/1
  mult_1/1 -> c1/1
  b1/1 -> mult_1/2
  a1/1 -> mult_1/1

== system xblocks_library_pfbs/pfb_fir/pfb_row_12/mult2 ==
  a1 : Inport
  b1 : Inport  Port=2
  a2 : Inport  Port=3
  b2 : Inport  Port=4
  mult_1 : xbsIndex_r4/Mult  precision=Full  arith_type="Signed  (2's comp)"  n_bits=16  bin_pt=14  quantization=Truncate  overflow=Wrap  en=off  latency=2  dbl_ovrd=off  use_behavioral_HDL=off  opt=Speed  use_embedded=on  optimum_pipeline=off  pipeline=on  use_rpm=on  placement_style=Triangular  block_type=mult
  mult_2 : xbsIndex_r4/Mult  precision=Full  arith_type="Signed  (2's comp)"  n_bits=16  bin_pt=14  quantization=Truncate  overflow=Wrap  en=off  latency=2  dbl_ovrd=off  use_behavioral_HDL=off  opt=Speed  use_embedded=on  optimum_pipeline=off  pipeline=on  use_rpm=on  placement_style=Triangular  block_type=mult
  c1 : Outport
  c2 : Outport  Port=2
  wires:
  mult_2/1 -> c2/1
  b2/1 -> mult_2/2
  a2/1 -> mult_2/1
  mult_1/1 -> c1/1
  b1/1 -> mult_1/2
  a1/1 -> mult_1/1

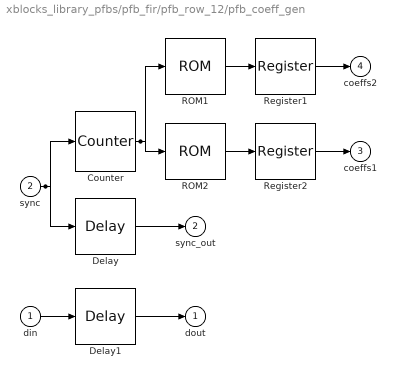
== system xblocks_library_pfbs/pfb_fir/pfb_row_12/pfb_coeff_gen ==
  din : Inport
  sync : Inport  Port=2
  Counter : xbsIndex_r4/Counter  cnt_type=Free Running  cnt_to=Inf  operation=Up  start_count=0  cnt_by_val=1  arith_type=Unsigned  n_bits=4  bin_pt=0  load_pin=off  rst=on  en=off  explicit_period=on  period=1  dbl_ovrd=off  use_behavioral_HDL=off  implementation=Fabric  use_rpm=on  block_type=counter
  Delay : xbsIndex_r4/Delay  en=off  latency=3  dbl_ovrd=off  reg_retiming=off  block_type=delay
  Delay1 : xbsIndex_r4/Delay  en=off  latency=3  dbl_ovrd=off  reg_retiming=off  block_type=delay
  ROM1 : xbsIndex_r4/ROM  depth=16  initVector=[0.0026501201486707 0.0102404214414259 0.0241890906187353 0.0484949792677442 0.0866786686039924 0.141225410855732 0.213113936374068 0.301496796003045 0.403581238821797 0.514736063656151 0.628822336302249 0.738717825898593 0.836980105084559 0.916574750769155 0.971585457997275 0.997823494908459]  distributed_mem=Block RAM  rst=off  init_reg=0  en=off  latency=2  arith_type="Signed  (2's comp)"  n_bits=18  bin_pt=17  dbl_ovrd=off  optimize=Area  use_rpm=on  block_type=sprom
  ROM2 : xbsIndex_r4/ROM  depth=16  initVector=[0.993264822418649 0.958263086338884 0.895513099914161 0.809769056143494 0.707350805829169 0.595496440858102 0.481637011666691 0.372677315570167 0.274364383314177 0.19081297621167 0.124236779165305 0.0749077778442863 0.0413379614417491 0.0206506376157481 0.00908666657559438 0.00257650165944676]  distributed_mem=Block RAM  rst=off  init_reg=0  en=off  latency=2  arith_type="Signed  (2's comp)"  n_bits=18  bin_pt=17  dbl_ovrd=off  optimize=Area  use_rpm=on  block_type=sprom
  Register1 : xbsIndex_r4/Register  init=0  rst=off  en=off  dbl_ovrd=off  block_type=register
  Register2 : xbsIndex_r4/Register  init=0  rst=off  en=off  dbl_ovrd=off  block_type=register
  dout : Outport
  sync_out : Outport  Port=2
  coeffs1 : Outport  Port=3
  coeffs2 : Outport  Port=4
  wires:
  sync/1 -> Delay/1, Counter/1
  Counter/1 -> ROM1/1, ROM2/1
  Register1/1 -> coeffs2/1
  ROM1/1 -> Register1/1
  Register2/1 -> coeffs1/1
  ROM2/1 -> Register2/1
  Delay1/1 -> dout/1
  din/1 -> Delay1/1
  Delay/1 -> sync_out/1

== system xblocks_library_pfbs/pfb_fir/pfb_row_12/ri_to_c0 ==
  re : Inport
  im : Inport  Port=2
  concat : xbsIndex_r4/Concat  num_inputs=2  dbl_ovrd=off  block_type=concat
  force_im : xbsIndex_r4/Reinterpret  force_arith_type=on  arith_type=Unsigned  force_bin_pt=on  bin_pt=0  block_type=reinterpret
      settings: infoedit="Changes signal type without altering the binary representation.   You can changed the signal between signed and unsigned, and relocate the binary point.<br><br>Hardware notes: In hardware this block costs nothing.<br><br>Example:  Suppose the input is 6 bits wide, signed, with 2 fractional bits, and the output is forced to unsigned with 0 fractional bits.  Then an input of -2.0 (1110.00 in binary 2's complement) becomes an output of 56 (111000 in binary)."
  force_re : xbsIndex_r4/Reinterpret  force_arith_type=on  arith_type=Unsigned  force_bin_pt=on  bin_pt=0  block_type=reinterpret
      settings: infoedit="Changes signal type without altering the binary representation.   You can changed the signal between signed and unsigned, and relocate the binary point.<br><br>Hardware notes: In hardware this block costs nothing.<br><br>Example:  Suppose the input is 6 bits wide, signed, with 2 fractional bits, and the output is forced to unsigned with 0 fractional bits.  Then an input of -2.0 (1110.00 in binary 2's complement) becomes an output of 56 (111000 in binary)."
  c : Outport
  wires:
  force_re/1 -> concat/1
  re/1 -> force_re/1
  force_im/1 -> concat/2
  im/1 -> force_im/1
  concat/1 -> c/1

== system xblocks_library_pfbs/pfb_fir/pfb_row_12/sync_delay ==
  In : Inport
  sync_del : xbsIndex_r4/Delay  en=off  latency=18  dbl_ovrd=off  reg_retiming=off  block_type=delay
  Out : Outport
  wires:
  sync_del/1 -> Out/1
  In/1 -> sync_del/1

== system xblocks_library_pfbs/pfb_fir/pfb_row_12/tap_split_1 ==
  inport : Inport
  Reinterp1 : xbsIndex_r4/Reinterpret  force_arith_type=on  arith_type="Signed  (2's comp)"  force_bin_pt=on  bin_pt=7  block_type=reinterpret
      settings: infoedit="Changes signal type without altering the binary representation.   You can changed the signal between signed and unsigned, and relocate the binary point.<br><br>Hardware notes: In hardware this block costs nothing.<br><br>Example:  Suppose the input is 6 bits wide, signed, with 2 fractional bits, and the output is forced to unsigned with 0 fractional bits.  Then an input of -2.0 (1110.00 in binary 2's complement) becomes an output of 56 (111000 in binary)."
  Reinterp2 : xbsIndex_r4/Reinterpret  force_arith_type=on  arith_type="Signed  (2's comp)"  force_bin_pt=on  bin_pt=7  block_type=reinterpret
      settings: infoedit="Changes signal type without altering the binary representation.   You can changed the signal between signed and unsigned, and relocate the binary point.<br><br>Hardware notes: In hardware this block costs nothing.<br><br>Example:  Suppose the input is 6 bits wide, signed, with 2 fractional bits, and the output is forced to unsigned with 0 fractional bits.  Then an input of -2.0 (1110.00 in binary 2's complement) becomes an output of 56 (111000 in binary)."
  Slice1 : xbsIndex_r4/Slice  nbits=8  boolean_output=off  mode=Upper Bit Location + Width  bit1=-0  base1=MSB of Input  bit0=0  base0=LSB of Input  dbl_ovrd=off  block_type=slice
  Slice2 : xbsIndex_r4/Slice  nbits=8  boolean_output=off  mode=Upper Bit Location + Width  bit1=-8  base1=MSB of Input  bit0=0  base0=LSB of Input  dbl_ovrd=off  block_type=slice
  outport1 : Outport
  outport2 : Outport  Port=2
  wires:
  inport/1 -> Slice2/1, Slice1/1
  Reinterp2/1 -> outport2/1
  Slice2/1 -> Reinterp2/1  "slice_out2"
  Reinterp1/1 -> outport1/1
  Slice1/1 -> Reinterp1/1  "slice_out1"

== system xblocks_library_pfbs/pfb_fir/pfb_row_12/tap_split_2 ==
  inport : Inport
  Reinterp1 : xbsIndex_r4/Reinterpret  force_arith_type=on  arith_type="Signed  (2's comp)"  force_bin_pt=on  bin_pt=7  block_type=reinterpret
      settings: infoedit="Changes signal type without altering the binary representation.   You can changed the signal between signed and unsigned, and relocate the binary point.<br><br>Hardware notes: In hardware this block costs nothing.<br><br>Example:  Suppose the input is 6 bits wide, signed, with 2 fractional bits, and the output is forced to unsigned with 0 fractional bits.  Then an input of -2.0 (1110.00 in binary 2's complement) becomes an output of 56 (111000 in binary)."
  Reinterp2 : xbsIndex_r4/Reinterpret  force_arith_type=on  arith_type="Signed  (2's comp)"  force_bin_pt=on  bin_pt=7  block_type=reinterpret
      settings: infoedit="Changes signal type without altering the binary representation.   You can changed the signal between signed and unsigned, and relocate the binary point.<br><br>Hardware notes: In hardware this block costs nothing.<br><br>Example:  Suppose the input is 6 bits wide, signed, with 2 fractional bits, and the output is forced to unsigned with 0 fractional bits.  Then an input of -2.0 (1110.00 in binary 2's complement) becomes an output of 56 (111000 in binary)."
  Slice1 : xbsIndex_r4/Slice  nbits=8  boolean_output=off  mode=Upper Bit Location + Width  bit1=-0  base1=MSB of Input  bit0=0  base0=LSB of Input  dbl_ovrd=off  block_type=slice
  Slice2 : xbsIndex_r4/Slice  nbits=8  boolean_output=off  mode=Upper Bit Location + Width  bit1=-8  base1=MSB of Input  bit0=0  base0=LSB of Input  dbl_ovrd=off  block_type=slice
  outport1 : Outport
  outport2 : Outport  Port=2
  wires:
  inport/1 -> Slice2/1, Slice1/1
  Reinterp2/1 -> outport2/1
  Slice2/1 -> Reinterp2/1  "slice_out2"
  Reinterp1/1 -> outport1/1
  Slice1/1 -> Reinterp1/1  "slice_out1"

== system xblocks_library_pfbs/pfb_fir/pfb_row_21/adder_tree1 ==
  sync : Inport
  din_1 : Inport  Port=2
  din_2 : Inport  Port=3
  adder_0 : xbsIndex_r4/AddSub  mode=Addition  use_carryin=off  use_carryout=off  en=off  latency=1  precision=Full  arith_type=Unsigned  n_bits=18  bin_pt=17  quantization="Round  (unbiased: +/- Inf)"  overflow=Wrap  dbl_ovrd=off  use_behavioral_HDL=on  hw_selection=Fabric  pipelined=off  block_type=addsub
  sync_delay : xbsIndex_r4/Delay  en=off  latency=1  dbl_ovrd=off  reg_retiming=off  block_type=delay
  sync_out : Outport
  dout : Outport  Port=2
  wires:
  adder_0/1 -> dout/1
  din_1/1 -> adder_0/2
  din_2/1 -> adder_0/1
  sync_delay/1 -> sync_out/1
  sync/1 -> sync_delay/1

== system xblocks_library_pfbs/pfb_fir/pfb_row_21/adder_tree2 ==
  sync : Inport
  din_1 : Inport  Port=2
  din_2 : Inport  Port=3
  adder_0 : xbsIndex_r4/AddSub  mode=Addition  use_carryin=off  use_carryout=off  en=off  latency=1  precision=Full  arith_type=Unsigned  n_bits=18  bin_pt=17  quantization="Round  (unbiased: +/- Inf)"  overflow=Wrap  dbl_ovrd=off  use_behavioral_HDL=on  hw_selection=Fabric  pipelined=off  block_type=addsub
  sync_delay : xbsIndex_r4/Delay  en=off  latency=1  dbl_ovrd=off  reg_retiming=off  block_type=delay
  sync_out : Outport
  dout : Outport  Port=2
  wires:
  adder_0/1 -> dout/1
  din_1/1 -> adder_0/2
  din_2/1 -> adder_0/1
  sync_delay/1 -> sync_out/1
  sync/1 -> sync_delay/1

== system xblocks_library_pfbs/pfb_fir/pfb_row_21/delay_bram2 ==
  din_1_1 : Inport
  Constant2 : xbsIndex_r4/Constant  arith_type=Boolean  const=1  n_bits=1  bin_pt=0  explicit_period=on  period=1  equ=P=C  opselect=C  inp2=PCIN>>17  opr=+  inp1=P  carry=CIN  dbl_ovrd=off  block_type=constant
  Counter : xbsIndex_r4/Counter  cnt_type=Count Limited  cnt_to=2  operation=Up  start_count=0  cnt_by_val=1  arith_type=Unsigned  n_bits=3  bin_pt=0  load_pin=off  rst=off  en=off  explicit_period=on  period=1  dbl_ovrd=off  use_behavioral_HDL=off  implementation=Fabric  use_rpm=0  block_type=counter
  bram1 : xbsIndex_r4/Single Port RAM  depth=8  initVector=0  distributed_mem=Block RAM  write_mode=Read Before Write  rst=off  init_reg=0  en=off  latency=4  dbl_ovrd=off  optimize=Area  use_rpm=off  block_type=spram
  dout_1_1 : Outport
  wires:
  bram1/1 -> dout_1_1/1
  Constant2/1 -> bram1/3
  din_1_1/1 -> bram1/2
  Counter/1 -> bram1/1
